simulink model "ce500_model"  (R2019b)
settings: Solver=VariableStepAuto  StartTime=0.0  StopTime=10.0  RelTol=1e-3
values from neighbouring files (symbols this model uses):
  A = [x_u,  x_a,  x_t,  0,    x_u_g,                       x_a_g,      0 ... (first row only)    [main.m]
  B = [x_d_e,   0,                                   0 ... (first row only)    [main.m]
  C = [C ... (first row only)    [main.m]
  D = [D ... (first row only)    [main.m]
settings Model: Creator=mauro  LastModifiedBy=mauro

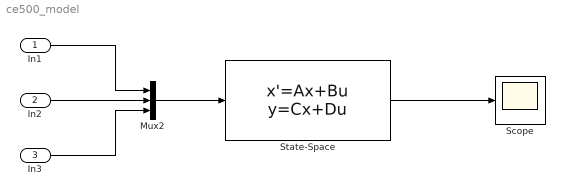
== system ce500_model ==
  In1 : Inport
  In2 : Inport  Port=2
  In3 : Inport  Port=3
  Mux2 : Mux  Inputs=3
  Scope : Scope
  State-Space : StateSpace  A=A  B=B  C=C  D=D  InitialCondition=0
  wires:
  State-Space/1 -> Scope/1
  Mux2/1 -> State-Space/1
  In3/1 -> Mux2/3
  In2/1 -> Mux2/2
  In1/1 -> Mux2/1
